simulink model "TrafficLightsim"  (R2024b)
settings: Solver=VariableStepAuto  StartTime=0.0  StopTime=inf  RelTol=1e-3
settings Model: Creator=Samuel  LastModifiedBy=Samuel

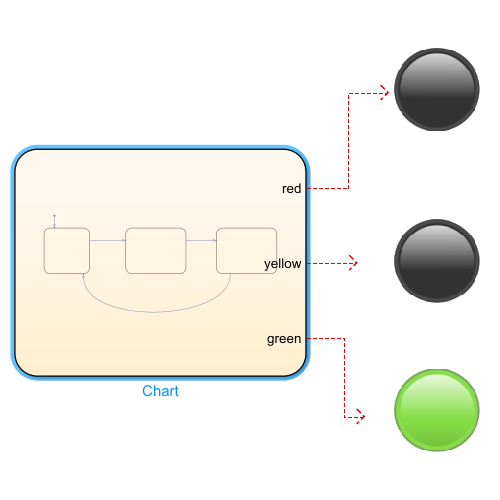
[thumbnail: Simulink's stored preview of the top-level diagram]
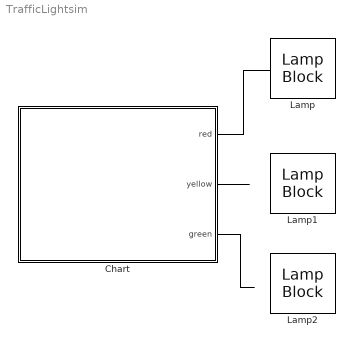
== system TrafficLightsim ==
  Chart : Stateflow chart  TreatAsAtomicUnit=on
  Lamp : LampBlock  LabelPosition=Hide
  Lamp1 : LampBlock  LabelPosition=Hide
  Lamp2 : LampBlock  LabelPosition=Hide
  wires:
  Chart/1(red) -> ?
  Chart/2(yellow) -> ?
  Chart/3(green) -> ?

== stateflow chart TrafficLightsim/Chart ==
  state red
    entry:
    red = false;
    yellow = true;
    green = true;
    exit:
    red = true;
  state yellow
    entry:
    red = true;
    yellow = false;
    green = true;
    exit:
    yellow = true;
  state green
    entry:
    red = true;
    yellow = true;
    green = false;
    exit:
    green = true;
  (default) -> red
  yellow -> green : after (3, sec)
  red -> yellow : after (10, sec)
  green -> red : after (30, sec)
  data: red output boolean size=1 =true; yellow output boolean size=1 =false; green output boolean size=1 =false
